simulink model "lab1simulink"  (R2019b)
settings: Solver=ode45  StartTime=0.0  StopTime=10.0  MaxStep=0.001  RelTol=1e-3
settings Model: Creator=wesle  LastModifiedBy=wesle
settings DataIOCC: ReturnWorkspaceOutputs=off

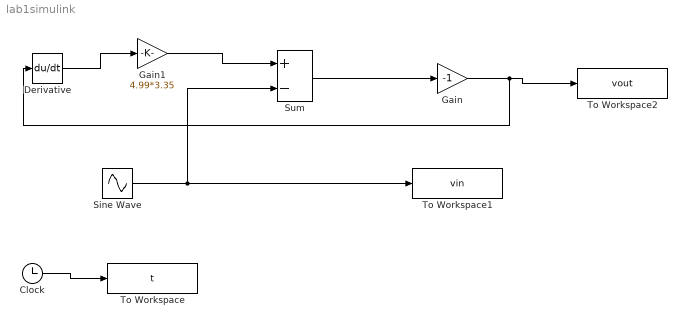
== system lab1simulink ==
  Clock : Clock
  Derivative : Derivative
  Gain : Gain  Gain=-1
  Gain1 : Gain  Gain=4.99*3.35
  Sine Wave : Sin  Frequency=2*pi  Phase=pi/2  SampleTime=0
  Sum : Sum  Inputs=+-
  To Workspace : ToWorkspace  VariableName=t  SampleTime=-1
  To Workspace1 : ToWorkspace  VariableName=vin  SampleTime=-1
  To Workspace2 : ToWorkspace  VariableName=vout  SampleTime=-1
  wires:
  Clock/1 -> To Workspace/1
  Sine Wave/1 -> Sum/2, To Workspace1/1
  Derivative/1 -> Gain1/1
  Gain1/1 -> Sum/1
  Sum/1 -> Gain/1
  Gain/1 -> Derivative/1, To Workspace2/1
